simulink model "doc_scalar_quant_1"  (Simulink 6.0)
settings: Solver=ode45  StartTime=0.0  StopTime=12  RelTol=1e-3
undefined symbols (not defined in the file): slcm
libraries: commsrccod2 x1, dspsrcs4 x1
settings Model: Creator=agaltman  LastModifiedBy=agaltman  ProdHWDeviceType=Specified
settings DataIOCC: SignalLoggingName=logsOut
settings OptimizationCC: BlockReduction=off  BooleanDataType=off  MultiInstanced=off
settings FormatCC: IgnoreBidirectionalLines=off
settings HardwareCC: ProdHWDeviceType=Specified
settings CodeAppCC: FileBanners=off  CustomSymbols=off  MangleLength=5
settings GRTTargetCC: TargetFcnLib=iso_c_tmw.mat  IsERTTarget=off

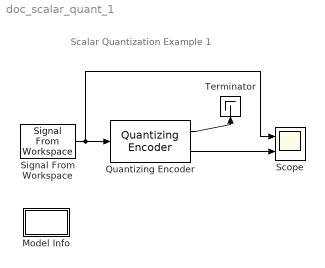
== system doc_scalar_quant_1 ==
  note: Scalar Quantization Example 1
  Model Info : Subsystem  LoadFcn=slcm LoadBlock;  InitFcn=slcm('UpdateAllCMBlocksInThisModelInit')  mask(CMBlock){InitialSaveTempField=, InitialBlockCM=none, BlockCM=none, Frame=on, SaveTempField=, DisplayStringWithTags=Info, MaskDisplayString=Info, HorizontalTextAlignment=Center, LeftAlignmentValue=0.5, SourceBlockDiagram=doc_scalar_quant_1, TagMaxNumber=20, CMTag1=, CMTag2=, CMTag3=, CMTag4=, CMTag5=, CMTag6=, CMTag7=, CMTag8=, CMTag9=, CMTag10=, CMTag11=, CMTag12=, CMTag13=, CMTag14=, CMTag15=, CMTag16=, CMTag17=, CMTag18=, CMTag19=, CMTag20=}
      mask help: This block allows revision control information to be displayed within the model.
      settings: CopyFcn=slcm CopyBlock;  DeleteFcn=slcm Cancel;  PostSaveFcn=slcm('UpdateAllCMBlocksInThisModel')  NameChangeFcn=slcm Rename;  OpenFcn=commdemohelp;
      mask Display: text(str2num(LeftAlignmentValue), 0.5, MaskDisplayString, 'HorizontalAlignment', HorizontalTextAlignment)
  Quantizing Encoder : commsrccod2/Quantizing Encoder  partition=[0,1,3]  codebook=[-1,.5,2,3]
  Scope : Scope  NumInputPorts=2
      settings: YMin=-2.6~-2.6  YMax=3.7~3.7
  Signal From Workspace : dspsrcs4/Signal From Workspace  X=[-2.4, -1, -.2, 0, .2, 1, 1.2, 1.9, 2, 2.9, 3, 3.5]'  Ts=1  nsamps=1  OutputAfterFinalValue=Setting to zero
  Terminator : Terminator
      settings: Orientation=up
  wires:
  Signal From Workspace/1 -> Scope/1, Quantizing Encoder/1
  Quantizing Encoder/1 -> Terminator/1
  Quantizing Encoder/2 -> Scope/2

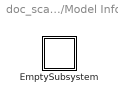
== system doc_scalar_quant_1/Model Info ==
  EmptySubsystem : Subsystem

== system doc_scalar_quant_1/Model Info/EmptySubsystem ==
